simulink model "DatacurationforN4SID"  (R2024b)
settings: Solver=VariableStepAuto  StartTime=0.0  StopTime=12  RelTol=1e-3
settings Model: Creator=shree  LastModifiedBy=shree

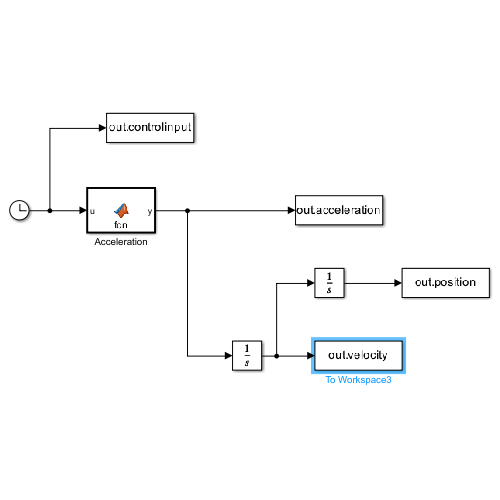
[thumbnail: Simulink's stored preview of the top-level diagram]
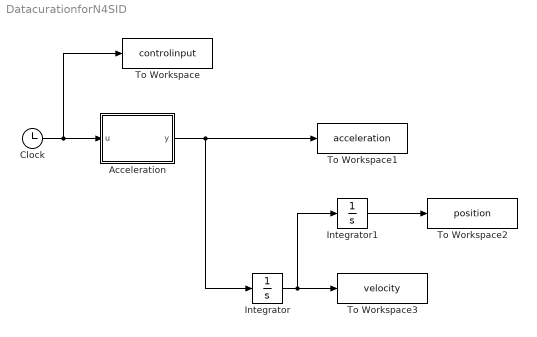
== system DatacurationforN4SID ==
  Acceleration : MATLAB Function  TreatAsAtomicUnit=on
  Clock : Clock
      settings: Decimation=12
  Integrator : Integrator
  Integrator1 : Integrator
  To Workspace : ToWorkspace  VariableName=controlinput  SampleTime=0.01
  To Workspace1 : ToWorkspace  VariableName=acceleration  SampleTime=0.01
  To Workspace2 : ToWorkspace  VariableName=position  SampleTime=0.01
  To Workspace3 : ToWorkspace  VariableName=velocity  SampleTime=0.01
  wires:
  Acceleration/1(y) -> To Workspace1/1, Integrator/1
  Integrator/1 -> To Workspace3/1, Integrator1/1
  Integrator1/1 -> To Workspace2/1
  Clock/1 -> To Workspace/1, Acceleration/1(u)

== matlab function DatacurationforN4SID/Acceleration ==
  data: u input; y output
function y = fcn(u)
    x = zeros(size(u)); 
    if all(u >= 0 & u <= 4)
        x(u >= 0 & u <= 4) = 2.5 * u(u >= 0 & u <= 4) - 10;
    elseif all(u > 4 & u < 7)
        x(u > 4 & u < 7) = 0;
    elseif all(u >= 7 & u <= 12)
        x(u >= 7 & u <= 12) = 2 * u(u >= 7 & u <= 12) - 14;
    end
    y = x;
end
